simulink model "longTransmissionLine"  (R2024b)
settings: Solver=VariableStepAuto  StartTime=0.0  StopTime=1.0  RelTol=1e-3
libraries: spsRMSLib x4, spsPower3phInstantaneousLib x2, spsThreePhaseVIMeasurementLib x2, spsDistributedParametersLineLib x1, spsThreePhaseSeriesRLCLoadLib x1, spsThreePhaseSourceLib x1, sps_lib x1
settings Model: Creator=ravit  LastModifiedBy=ravit

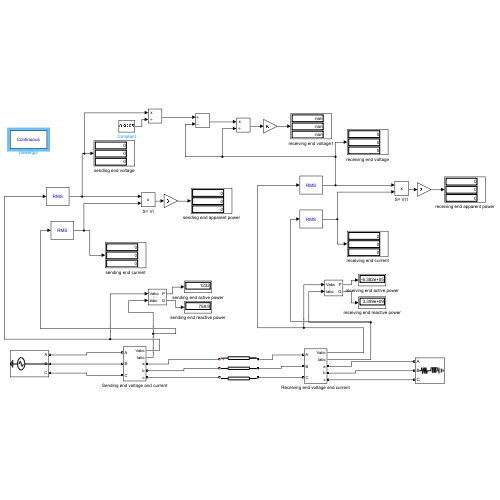
[thumbnail: Simulink's stored preview of the top-level diagram]
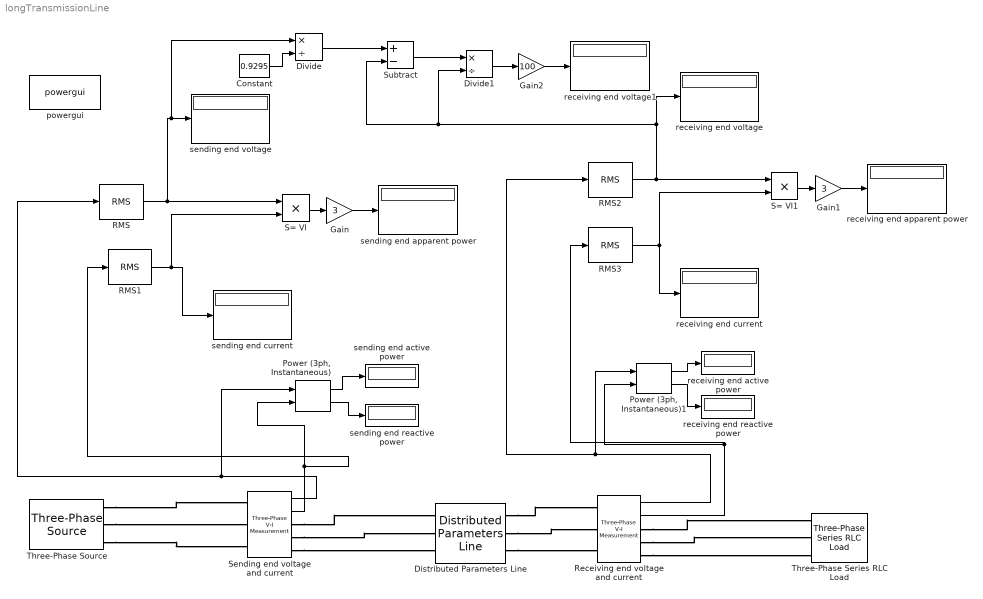
== system longTransmissionLine ==
  Constant : Constant  Value=0.9295
  Distributed Parameters Line : spsDistributedParametersLineLib/Distributed Parameters Line  Phases=3  Length=300  Frequency=60  Resistance=[0 0]  Inductance="[0.97e-3  0.99e-3]"  Capacitance=[11.5e-9 11.5e-9]  x1=[5.82076609134674e-11 617530 617530;376.991118430775 376.991118430775 376.991118430775;1.18918707880175 0.426861843081656 -1.14393448371324]  x2=[1.54333976486453e-10 1.44117594092296e-06 1.44135076949553e-06;376.991118430775 376.991118430775 376.991118430775;0.421294429503861 -0.50037378567285 -2.07126077139894]  x3=[1.45590189218475e-12 5765.15930898519 5765.15930898519;376.991118430775 376.991118430775 376.991118430775;-1.27766463256449 1.61992322779004 0.0491269009951449]  x4=[8.19807445501281e-13 5765.15930899313 5765.15930899313;376.991118430775 376.991118430775 376.991118430775;0.601184475254179 -1.14393448371099 -2.71473081050589]  x5=0.00101224996912818  V1=[5.821e-11 6.175e+05 6.175e+05;377 377 377;1.189 0.4269 -1.144]  V2=[1.543e-10 1.441e-06 1.441e-06;377 377 377;0.4213 -0.5004 -2.071]  I1=[1.456e-12 5765 5765;377 377 377;-1.278 1.62 0.04913]  I2=[8.198e-13 5765 5765;377 377 377;0.6012 -1.144 -2.715]  nHarmo=1  Measurements=None  Decoupling=off  VsMag0=0  VrMag0=0  VsAngle0=0  VrAngle0=0  IsMag0=0  IrMag0=0  IsAngle0=0  IrAngle0=0
      settings: LibrarySourceBlock=sps_lib/Power Grid Elements/Distributed Parameters Line
  Divide : Product  Inputs=*/
  Divide1 : Product  Inputs=*/
  Gain : Gain  Gain=3
  Gain1 : Gain  Gain=3
  Gain2 : Gain  Gain=100
  "Power (3ph, Instantaneous)" : spsPower3phInstantaneousLib/Power (3ph, Instantaneous)
  "Power (3ph, Instantaneous)1" : spsPower3phInstantaneousLib/Power (3ph, Instantaneous)
  RMS{,1..3} (4 alike) : spsRMSLib/RMS  TrueRMS=on  Freq=60  RMSInit=0  Ts=0
  Receiving end voltage and current : spsThreePhaseVIMeasurementLib/Three-Phase V-I Measurement  VoltageMeasurement=phase-to-ground  SetLabelV=off  LabelV=Vabc  Vpu=off  VpuLL=off  CurrentMeasurement=yes  SetLabelI=off  LabelI=Iabc  Ipu=off  Pbase=100e6  Vbase=500e3  OutputType=Complex  PhasorSimulation=off  PSBequivalent=0
  S= VI : Product
  S= VI1 : Product
  Sending end voltage and current : spsThreePhaseVIMeasurementLib/Three-Phase V-I Measurement  VoltageMeasurement=phase-to-ground  SetLabelV=off  LabelV=Vabc  Vpu=off  VpuLL=off  CurrentMeasurement=yes  SetLabelI=off  LabelI=Iabc  Ipu=off  Pbase=100e6  Vbase=500e3  OutputType=Complex  PhasorSimulation=off  PSBequivalent=0
  Subtract : Sum  Inputs=+-
  Three-Phase Series RLC Load : spsThreePhaseSeriesRLCLoadLib/Three-Phase Series RLC Load  LConnTagsString=A|B|C  Configuration=Y (grounded)  NominalVoltage=500e-3  Vabc=[1e3 1e3 1e3]  Vabcp=[1e3 1e3 1e3]  NominalFrequency=60  UnbalancedPower=off  ActivePower=800e6  InductivePower=600e6  CapacitivePower=0  Pabc=[10e3 9e3 11e3]  QLabc=[100 90 110]  QCabc=[100 90 110]  Pabcp=[10e3 9e3 11e3]  QLabcp=[100 90 110]  QCabcp=[100 90 110]  Measurements=None  LoadType=constant Z
  Three-Phase Source : spsThreePhaseSourceLib/Three-Phase Source  InternalConnection=Yg  VoltagePhases=off  Voltage=617.53e3  PhaseAngle=16.1  Voltage_phases=[25e3 25e3 25e3]/sqrt(3)  PhaseAngles_phases=[0 -120 +120]  Frequency=60  NonIdealSource=off  SpecifyImpedance=off  Resistance=0.8929  Inductance=16.58e-3  ShortCircuitLevel=100e6  BaseVoltage=25e3  XRratio=7  BusType=swing  Pref=10e3  Qref=0  Prefabc=[10e3, 10e3, 10e3]  Qrefabc=[0, 0, 0]  Qmin=-inf  Qmax=inf
  powergui : sps_lib/powergui  Priority=1  SimulationMode=Continuous  SampleTime=50e-6  frequency=60  Iterations=50  frequencyindice=60  Pbase=100e6  ErrMax=1e-4  UnitsV=kV  UnitsW=MW  buscounter=0  FunctionMessages=off  echomessages=off  EnableUseOfTLC=off  CurrentSourceSwitches=off  DisableSnubberDevices=off  DisableRonSwitches=off  DisableVfSwitches=off  DisplayEquations=off  AutomaticDiscreteSolvers=off  SolverType=Tustin/Backward Euler (TBE)  Interpol=off  ExternalGateDelay=off  methode=off  Ts=100  x0status=blocks  SPID=on  SwTol=0  HookPort=off  NonlinearTolerance=1e-4  nMaxIteration=100  ContinueOnMaxIteration=off  RestoreLinks=warning  ResistiveCurrentMeasurement=off  Frange=[0:2:500]  Ylog=off  Xlog=on  ShowGrid=off  save=off  variable=ZData  structure=0  ZoomFFT=off  StartTime=0.0  cycles=1  DisplayStyle=1  fundamental=60  FreqAxis=off  MaxFrequency=1000  frequencyindicesteady=1  RmsSteady=1  display=off
  receiving end active power : Display
  receiving end apparent power : Display
  receiving end current : Display
  receiving end reactive power : Display
  receiving end voltage : Display
  receiving end voltage1 : Display
  sending end active power : Display
  sending end apparent power : Display
  sending end current : Display
  sending end reactive power : Display
  sending end voltage : Display
  wires:
  Sending end voltage and current/1 -> "Power (3ph, Instantaneous)"/1, RMS/1
  RMS/1 -> Divide/1, sending end voltage/1, S= VI/1
  RMS1/1 -> S= VI/2, sending end current/1
  Sending end voltage and current/2 -> "Power (3ph, Instantaneous)"/2, RMS1/1
  "Power (3ph, Instantaneous)"/1 -> sending end active power/1
  "Power (3ph, Instantaneous)"/2 -> sending end reactive power/1
  S= VI/1 -> Gain/1
  Gain/1 -> sending end apparent power/1
  "Power (3ph, Instantaneous)1"/1 -> receiving end active power/1
  "Power (3ph, Instantaneous)1"/2 -> receiving end reactive power/1
  Gain1/1 -> receiving end apparent power/1
  RMS2/1 -> Divide1/2, Subtract/2, receiving end voltage/1, S= VI1/1
  Receiving end voltage and current/2 -> RMS3/1, "Power (3ph, Instantaneous)1"/2
  Receiving end voltage and current/1 -> "Power (3ph, Instantaneous)1"/1, RMS2/1
  RMS3/1 -> S= VI1/2, receiving end current/1
  S= VI1/1 -> Gain1/1
  Constant/1 -> Divide/2
  Divide/1 -> Subtract/1
  Subtract/1 -> Divide1/1
  Divide1/1 -> Gain2/1
  Gain2/1 -> receiving end voltage1/1
  connections:
  Three-Phase Source/RConn1 -- Sending end voltage and current/LConn1
  Three-Phase Source/RConn2 -- Sending end voltage and current/LConn2
  Three-Phase Source/RConn3 -- Sending end voltage and current/LConn3
  Sending end voltage and current/RConn3 -- Distributed Parameters Line/LConn3
  Sending end voltage and current/RConn2 -- Distributed Parameters Line/LConn2
  Sending end voltage and current/RConn1 -- Distributed Parameters Line/LConn1
  Distributed Parameters Line/RConn1 -- Receiving end voltage and current/LConn1
  Distributed Parameters Line/RConn2 -- Receiving end voltage and current/LConn2
  Distributed Parameters Line/RConn3 -- Receiving end voltage and current/LConn3
  Receiving end voltage and current/RConn1 -- Three-Phase Series RLC Load/LConn1
  Receiving end voltage and current/RConn2 -- Three-Phase Series RLC Load/LConn2
  Receiving end voltage and current/RConn3 -- Three-Phase Series RLC Load/LConn3
